simulink model "sysid_cat"  (R2017b)
settings: Solver=FixedStepAuto  StartTime=0.0  StopTime=inf  FixedStep=0.02  RelTol=1e-3
undefined symbols (not defined in the file): Angular, Linear
libraries: robotlib x6
settings Model: Creator=ece446  LastModifiedBy=ece446
settings SolverCC: AlgebraicLoopSolver=LineSearch
settings OptimizationCC: PassReuseOutputArgsAs=Individual arguments  MaxStackSize=64
settings DebuggingCC: ParameterTunabilityLossMsg=error
settings HardwareCC: ProdBitPerPointer=32  ProdBitPerSizeT=32  ProdBitPerPtrDiffT=32  ProdLargestAtomicFloat=None  ProdWordSize=32  ProdHWDeviceType=Custom Processor->Custom
settings SFSimCC: MATLABDynamicMemAlloc=off
settings RTWCC: SystemTargetFile=ert.tlc  HardwareBoard=Robot Operating System (ROS)  TemplateMakefile=ert_default_tmf  GenerateReport=on  Toolchain=Catkin  IncludeHyperlinkInReport=on  LaunchReport=on  TargetLang=C++  GenerateTraceInfo=on  GenerateTraceReport=on  GenerateTraceReportSl=on  GenerateTraceReportSf=on  GenerateTraceReportEml=on
settings CodeAppCC: ForceParamTrailComments=on  IgnoreCustomStorageClasses=off  OperatorAnnotations=on  SimulinkDataObjDesc=on  SFDataObjDesc=on  InsertBlockDesc=on

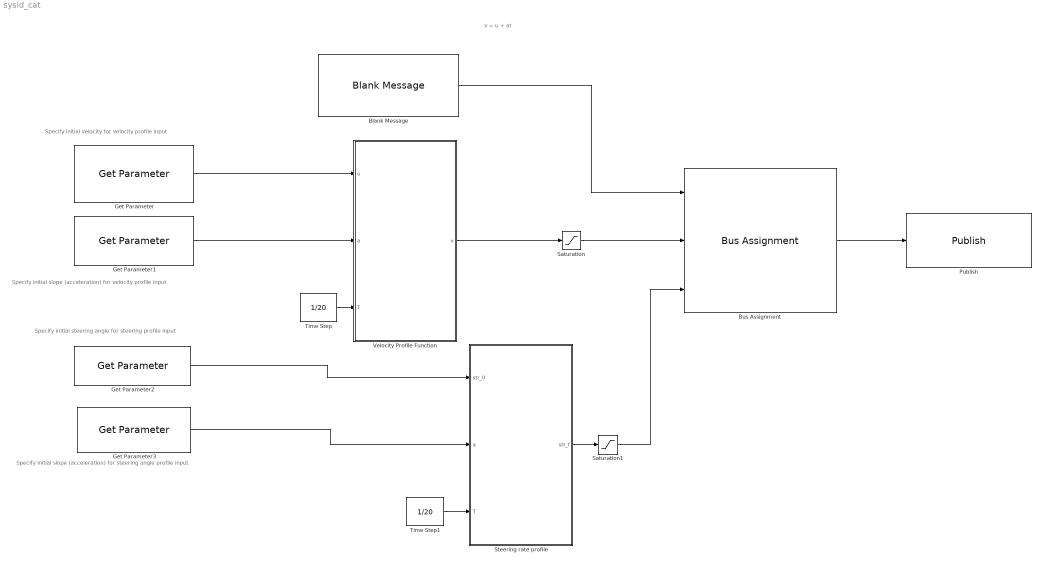
== system sysid_cat ==
  note: v = u + at
  note: Specify initial velocity for velocity profile input
  note: Specify initial slope (acceleration) for velocity profile input
  note: Specify initial steering angle for steering profile input
  note: Specify initial slope (acceleration) for steering angle profile input
  Blank Message : robotlib/Blank Message  SourceLibraryInfo=This block requires Robotics System Toolbox  messageType=geometry_msgs/Twist  SampleTime=inf
      settings: SourceProductBaseCode=RO
  Bus Assignment : BusAssignment  AssignedSignals=Linear.X,Angular.Z
  Get Parameter : robotlib/Get Parameter  SourceLibraryInfo=This block requires Robotics System Toolbox  ParameterSource=Specify your own  ParameterName=init_vel  ParameterType=double  ParameterMaxArrayLength=16  ParameterInitialValue=0.1  SampleTime=-1  ShowErrorCodeOutput=off  ModelName=sysid_cat  BlockId=ParamGet_sysid_cat_1
      settings: SourceProductName=Robotics System Toolbox  SourceProductBaseCode=RO
  Get Parameter1 : robotlib/Get Parameter  SourceLibraryInfo=This block requires Robotics System Toolbox  ParameterSource=Specify your own  ParameterName=vel_slope  ParameterType=double  ParameterMaxArrayLength=16  ParameterInitialValue=0.01  SampleTime=-1  ShowErrorCodeOutput=off  ModelName=sysid_cat  BlockId=ParamGet_sysid_cat_3
      settings: SourceProductName=Robotics System Toolbox  SourceProductBaseCode=RO
  Get Parameter2 : robotlib/Get Parameter  SourceLibraryInfo=This block requires Robotics System Toolbox  ParameterSource=Specify your own  ParameterName=init_str  ParameterType=double  ParameterMaxArrayLength=16  ParameterInitialValue=0.01  SampleTime=-1  ShowErrorCodeOutput=off  ModelName=sysid_cat  BlockId=ParamGet_sysid_cat_5
      settings: SourceProductName=Robotics System Toolbox  SourceProductBaseCode=RO
  Get Parameter3 : robotlib/Get Parameter  SourceLibraryInfo=This block requires Robotics System Toolbox  ParameterSource=Specify your own  ParameterName=str_slope  ParameterType=double  ParameterMaxArrayLength=16  ParameterInitialValue=0  SampleTime=-1  ShowErrorCodeOutput=off  ModelName=sysid_cat  BlockId=ParamGet_sysid_cat_6
      settings: SourceProductName=Robotics System Toolbox  SourceProductBaseCode=RO
  Publish : robotlib/Publish  SourceLibraryInfo=This block requires Robotics System Toolbox  topicSource=Specify your own  topic=cmd_vel  messageType=geometry_msgs/Twist  messageQueueLength=1
      settings: SourceProductBaseCode=RO
  Saturation : Saturate  UpperLimit=32  LowerLimit=0
  Saturation1 : Saturate  UpperLimit=0.6  LowerLimit=-0.6
  Steering rate profile : MATLAB Function  TreatAsAtomicUnit=on
  Time Step : Constant  Value=1/20
  Time Step1 : Constant  Value=1/20
  Velocity Profile Function : MATLAB Function  TreatAsAtomicUnit=on
  wires:
  Time Step/1 -> Velocity Profile Function/3(T)
  Get Parameter1/1 -> Velocity Profile Function/2(a)
  Get Parameter/1 -> Velocity Profile Function/1(u)
  Velocity Profile Function/1(v) -> Saturation/1
  Steering rate profile/1(str_f) -> Saturation1/1
  Get Parameter2/1 -> Steering rate profile/1(str_0)
  Get Parameter3/1 -> Steering rate profile/2(a)
  Time Step1/1 -> Steering rate profile/3(T)
  Blank Message/1 -> Bus Assignment/1
  Bus Assignment/1 -> Publish/1
  Saturation/1 -> Bus Assignment/2
  Saturation1/1 -> Bus Assignment/3

== matlab function sysid_cat/Steering rate profile ==
  data: str_0 input; str_f output; a input; T input
function str_f = velprofile(str_0, a, T)
persistent t
if isempty(t)
    t = T;
else
    t = t+T;
end

str_f = str_0 + a*t;

== matlab function sysid_cat/Velocity Profile Function ==
  data: u input; v output; a input; T input
function v = velprofile(u, a, T)
persistent t
if isempty(t)
    t = T;
else
    t = t+T;
end

v = u + a*t;
